simulink model "turn180"  (R2023a)
settings: Solver=FixedStepDiscrete  StartTime=0.0  StopTime=15  FixedStep=0.01  RelTol=1e-3
undefined symbols (not defined in the file or in its folder): InputPWM, WheelSpeed
libraries: mobileRoboticsTrainingLib x5, slpidlib x1
settings Model: Creator=Boitumelo  LastModifiedBy=Nate
settings DebuggingCC: UnconnectedInputMsg=warning  UnconnectedOutputMsg=warning  UnconnectedLineMsg=warning
settings ModelReferenceCC: EnableRefExpFcnMdlSchedulingChecks=on
settings RTWCC: DLArmComputeVersion=19.05

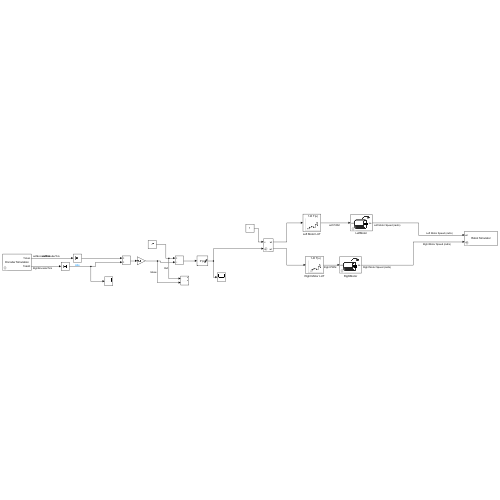
[thumbnail: Simulink's stored preview of the top-level diagram]
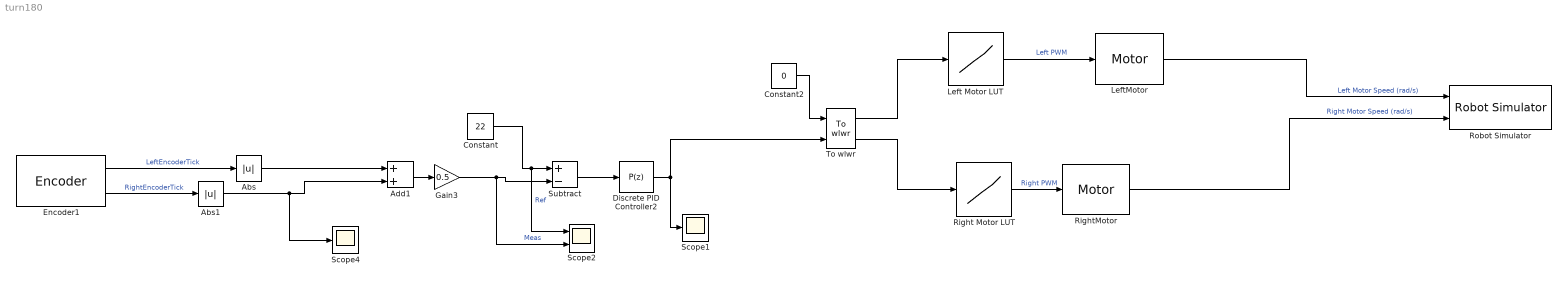
== system turn180 ==
  Abs : Abs  SaturateOnIntegerOverflow=off
  Abs1 : Abs  SaturateOnIntegerOverflow=off
  Add1 : Sum
  Constant : Constant  Value=22
  Constant2 : Constant  Value=0
  Discrete PID Controller2 : slpidlib/PID Controller  Controller=P  Form=Parallel  TimeDomain=Discrete-time  UseExternalTs=off  SampleTime=-1  IntegratorMethod=Forward Euler  FilterMethod=Forward Euler  ControllerParametersSource=internal  P=0.5  I=0.2  UseKiTs=off  D=0.4  N=50  UseFilter=on  TunerSelectOption=Transfer Function Based (PID Tuner App)  InitialConditionSource=internal  InitialConditionForIntegrator=0  InitialConditionForFilter=0  DifferentiatorICPrevScaledInput=0  ExternalReset=none  TrackingMode=off  Kt=1  LimitOutput=on  SatLimitsSource=internal  UpperSaturationLimit=0.32  LowerSaturationLimit=-0.32  LinearizeAsGain=off  AntiWindupMode=clamping  Kb=1  LimitIntegrator=off  UpperIntegratorSaturationLimit=inf  LowerIntegratorSaturationLimit=-inf  POutMin=[]  POutMax=[]  IOutMin=[]  IOutMax=[]  DOutMin=[]  DOutMax=[]  NOutMin=[]  NOutMax=[]  SumOutMin=[]  SumOutMax=[]  SaturationOutMin=[]  SaturationOutMax=[]  PParamMin=[]  PParamMax=[]  IParamMin=[]  IParamMax=[]  DParamMin=[]  DParamMax=[]  NParamMin=[]  NParamMax=[]  KbParamMin=[]  KbParamMax=[]  KtParamMin=[]  KtParamMax=[]  KbOutMin=[]  KbOutMax=[]  KtOutMin=[]  KtOutMax=[]  IntegratorOutMin=[]  IntegratorOutMax=[]  FilterOutMin=[]  FilterOutMax=[]  SumI1OutMin=[]  SumI1OutMax=[]  SumI2OutMin=[]  SumI2OutMax=[]  SumI3OutMin=[]  SumI3OutMax=[]  SumI4OutMin=[]  SumI4OutMax=[]  SumDOutMin=[]  SumDOutMax=[]  DifferentiatorOutMin=[]  DifferentiatorOutMax=[]  FilterDiffOutCoefMin=[]  FilterDiffOutCoefMax=[]  ReciprocalOutMin=[]  ReciprocalOutMax=[]  SumDenOutMin=[]  SumDenOutMax=[]  SumNumOutMin=[]  SumNumOutMax=[]  DivideOutMin=[]  DivideOutMax=[]  UdiffTsProdOutMin=[]  UdiffTsProdOutMax=[]  NTsProdOutMin=[]  NTsProdOutMax=[]  UintegralTsProdOutMin=[]  UintegralTsProdOutMax=[]  UngainTsProdOutMin=[]  UngainTsProdOutMax=[]  ClampingZeroOutDataTypeStr=Inherit: Inherit via back propagation  ClampingZeroOutMin=[]  ClampingZeroOutMax=[]  FilterDenConstantOutDataTypeStr=Inherit: Inherit via back propagation  FilterDenConstantOutMin=[]  FilterDenConstantOutMax=[]  PCopyOutDataTypeStr=Inherit: Inherit via back propagation  PCopyOutMin=[]  PCopyOutMax=[]  NCopyOutDataTypeStr=Inherit: Inherit via back propagation  NCopyOutMin=[]  NCopyOutMax=[]  IntegratorContinuousStateAttributes=''  IntegratorStateMustResolveToSignalObject=off  IntegratorRTWStateStorageClass=Auto  FilterContinuousStateAttributes=''  FilterStateMustResolveToSignalObject=off  FilterRTWStateStorageClass=Auto  ParallelPVariant=InternalParameters  IdealPVariant=Disabled  IVariant=Disabled  DVariant=Disabled  IntegratorVariant=Disabled  SatVariant=Enabled  AWVariant=Disabled  PCopyVariant=Disabled  TRVariant=Disabled  FdbkBlocksVariant=Forward  IdealPFdbkVariant=Disabled  SatFdbkVariant=Disabled  DerivativeFilterVariant=Disabled  NVariant=Disabled  NCopyVariant=Disabled_SignalSpec  FilterICVariant=Disabled  IntegratorICVariant=Disabled  ExternalResetVariant=Disabled  TRSumVariant=Passthrough  SumFdbkVariant=Disabled  SumVariant=Passthrough_P  TsampFilterVariant=InternalTs  TsampNgainVariant=Passthrough  TsampIntegralVariant=Disabled_SignalSpec  ExternalSaturationOutDataTypeStr=Inherit: Same as second input
      settings: LibrarySourceBlock=simulink/Discrete/Discrete PID Controller
  Encoder1 : mobileRoboticsTrainingLib/Encoder  axleLength=axleLength  wheelR=wheelR  ticksPerRot=ticksPerRot
      settings: SourceProductName=Mobile Robotics Training Library
  Gain3 : Gain  Gain=0.5
  Left Motor LUT : Lookup_n-D  NumberOfTableDimensions=1  BreakpointsForDimension1=WheelSpeed  Table=InputPWM  InterpMethod=Nearest  ExtrapMethod=Clip  InternalRulePriority=Speed  RndMeth=Simplest
  LeftMotor : mobileRoboticsTrainingLib/Motor  motorPlant=wheelMotorModel  sensorType=Speed
      settings: SourceProductName=Mobile Robotics Training Library
  Right Motor LUT : Lookup_n-D  NumberOfTableDimensions=1  BreakpointsForDimension1=WheelSpeed  Table=InputPWM  InterpMethod=Nearest  ExtrapMethod=Clip  InternalRulePriority=Speed  RndMeth=Simplest
  RightMotor : mobileRoboticsTrainingLib/Motor  motorPlant=wheelMotorModel  sensorType=Speed
      settings: SourceProductName=Mobile Robotics Training Library
  Robot Simulator : mobileRoboticsTrainingLib/Robot Simulator  Priority=99  mapVar=mapForSim  startX=0.5  startY=0.2  startTheta=90  axleLength=axleLength  wheelR=wheelR
  Scope1 : Scope
  Scope2 : Scope  NumInputPorts=2
  Scope4 : Scope
  Subtract : Sum  Inputs=+-
  To wlwr : mobileRoboticsTrainingLib/To wlwr  axleLength=axleLength  wheelR=wheelR
  wires:
  Right Motor LUT/1 -> RightMotor/1  "Right PWM"
  Left Motor LUT/1 -> LeftMotor/1  "Left PWM"
  To wlwr/1 -> Left Motor LUT/1
  To wlwr/2 -> Right Motor LUT/1
  RightMotor/1 -> Robot Simulator/2  "Right Motor Speed (rad/s)"
  LeftMotor/1 -> Robot Simulator/1  "Left Motor Speed (rad/s)"
  Constant2/1 -> To wlwr/1
  Encoder1/2 -> Abs1/1  "RightEncoderTick"
  Encoder1/1 -> Abs/1  "LeftEncoderTick"
  Add1/1 -> Gain3/1
  Gain3/1 -> Scope2/2, Subtract/2  "Meas"
  Constant/1 -> Scope2/1, Subtract/1  "Ref"
  Subtract/1 -> Discrete PID Controller2/1
  Discrete PID Controller2/1 -> To wlwr/2, Scope1/1
  Abs/1 -> Add1/1
  Abs1/1 -> Add1/2, Scope4/1
